simulink model "QPSK"  (R2020a)
settings: Solver=VariableStepAuto  StartTime=0.0  StopTime=200  RelTol=1e-3
libraries: simulink x7, dspsigops x2, commchan3 x1, dspstat3 x1, dspsrcs4 x1
settings Model: Creator=cxp10  LastModifiedBy=cxp10

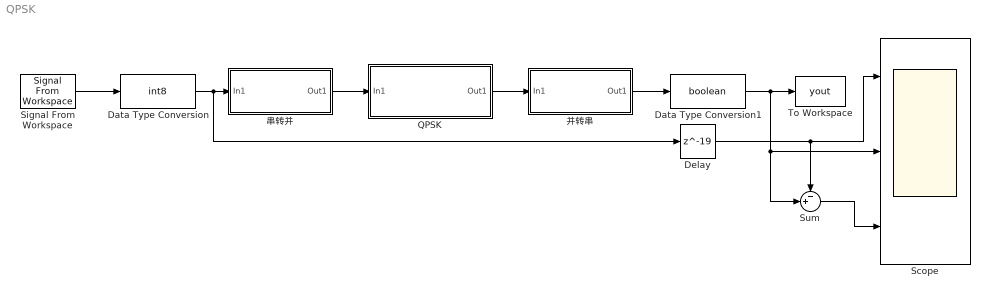
== system QPSK ==
  Data Type Conversion : DataTypeConversion  OutDataTypeStr=int8
  Data Type Conversion1 : DataTypeConversion  OutDataTypeStr=boolean
  Delay : Delay  DelayLength=19  InitialCondition=0  SampleTime=0.05
  QPSK : Subsystem
  Scope : Scope  NumInputPorts=3
  Signal From Workspace : dspsrcs4/Signal From Workspace  X=simin  Ts=0.05  nsamps=1  OutputAfterFinalValue=Setting to zero  ignoreOrWarnInputAndFrameLengths=off  OutputFrames=off
  Sum : Sum  Inputs=-+|
  To Workspace : ToWorkspace  VariableName=yout  SampleTime=-1
      settings: Save2DSignal=2-D array (concatenate along first dimension)
  串转并 : Subsystem
  并转串 : Subsystem
  wires:
  Data Type Conversion1/1 -> Sum/2, Scope/2, To Workspace/1
  Signal From Workspace/1 -> Data Type Conversion/1
  Sum/1 -> Scope/3
  并转串/1(Out1) -> Data Type Conversion1/1
  QPSK/1(Out1) -> 并转串/1(In1)
  串转并/1(Out1) -> QPSK/1(In1)
  Delay/1 -> Scope/1, Sum/1
  Data Type Conversion/1 -> 串转并/1(In1), Delay/1

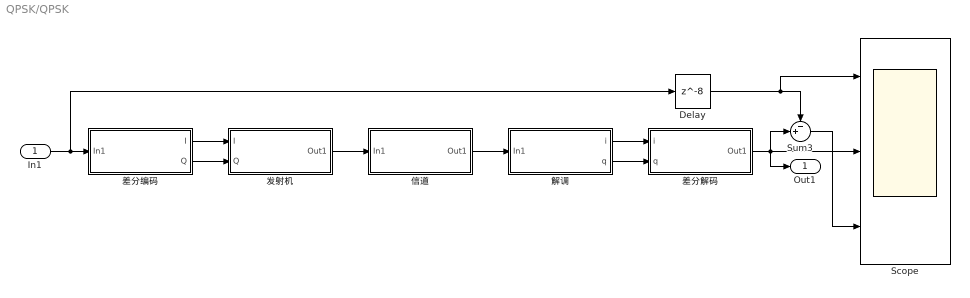
== system QPSK/QPSK ==
  In1 : Inport
  Delay : Delay  DelayLength=8  InitialCondition=0  SampleTime=0.1
  Scope : Scope  NumInputPorts=3
  Sum3 : Sum  Inputs=-+|
  信道 : Subsystem
  发射机 : Subsystem
  差分编码 : Subsystem
  差分解码 : Subsystem
  解调 : Subsystem
  Out1 : Outport
  wires:
  Delay/1 -> Sum3/1, Scope/1
  发射机/1(Out1) -> 信道/1(In1)
  解调/1(i) -> 差分解码/1(i)
  解调/2(q) -> 差分解码/2(q)
  信道/1(Out1) -> 解调/1(In1)
  Sum3/1 -> Scope/3
  差分编码/1(I) -> 发射机/1(I)
  差分编码/2(Q) -> 发射机/2(Q)
  In1/1 -> 差分编码/1(In1), Delay/1
  差分解码/1(Out1) -> Out1/1, Sum3/2, Scope/2

== system QPSK/串转并 ==
  In1 : Inport
  Delay : Delay  DelayLength=1  InitialCondition=0  SampleTime=0.05
  Delay1 : Delay  DelayLength=1  InitialCondition=0  SampleTime=0.1
  Gain : Gain  Gain=2
  Sum : Sum  Inputs=|++
  Out1 : Outport
  wires:
  Delay1/1 -> Out1/1
  Sum/1 -> Delay1/1
  In1/1 -> Sum/2, Delay/1
  Delay/1 -> Gain/1
  Gain/1 -> Sum/1

== system QPSK/并转串 ==
  In1 : Inport
  Counter Limited : simulink/Sources/Counter Limited  uplimit=1  tsamp=0.05
  Data Type Conversion : DataTypeConversion  OutDataTypeStr=fixdt(0,2,0)
  Extract Bits : simulink/Logic and Bit Operations/Extract Bits  bitsToExtract=Upper half  numBits=8  bitIdxRange=[0 7]  outScalingMode=Treat bit field as an integer
  Extract Bits1 : simulink/Logic and Bit Operations/Extract Bits  bitsToExtract=Lower half  numBits=8  bitIdxRange=[0 7]  outScalingMode=Treat bit field as an integer
  Switch : Switch  Criteria=u2 > Threshold
  Out1 : Outport
  wires:
  Extract Bits/1 -> Switch/3
  In1/1 -> Data Type Conversion/1
  Extract Bits1/1 -> Switch/1
  Data Type Conversion/1 -> Extract Bits1/1, Extract Bits/1
  Counter Limited/1 -> Switch/2
  Switch/1 -> Out1/1

== system QPSK/QPSK/信道 ==
  In1 : Inport
  AWGN Channel : commchan3/AWGN Channel  InputProcessing=Columns as channels (frame based)  seed=67  noiseMode="Signal to noise ratio  (SNR)"  EbNodB=10  EsNodB=10  SNRdB=5  bitsPerSym=1  Ps=0.0504  Tsym=1  variance=1
  Data Type Conversion : DataTypeConversion  OutDataTypeStr=double
  Data Type Conversion1 : DataTypeConversion
  Data Type Conversion2 : DataTypeConversion  OutDataTypeStr=fixdt(1,32,28)
  Mean : dspstat3/Mean  run=on  reset_popup=None  directionMode=Each column  dimension=1  roiEnable=off  roiType=Rectangles  roiPortion=Entire ROI  roiOutput=Individual statistics for each ROI  roiFlag=off  roundingMode=Floor  overflowMode=off  outputDataTypeStr=Inherit: Same as accumulator  outputMin=[]  outputMax=[]  outputLastDataTypeStr=Inherit: Same as accumulator
  Product : Product
  Scope1 : Scope
  Out1 : Outport
  wires:
  In1/1 -> Data Type Conversion/1
  AWGN Channel/1 -> Data Type Conversion2/1
  Data Type Conversion/1 -> Data Type Conversion1/1, AWGN Channel/1
  Product/1 -> Mean/1
  Data Type Conversion1/1 -> Product/2, Product/1
  Mean/1 -> Scope1/1
  Data Type Conversion2/1 -> Out1/1

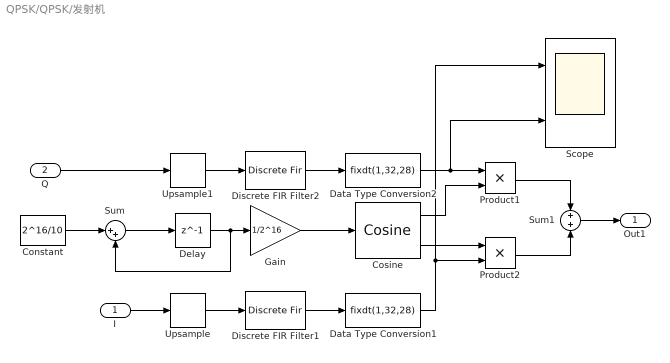
== system QPSK/QPSK/发射机 ==
  I : Inport
  Q : Inport  Port=2
  Constant : Constant  Value=2^16/10
  Cosine : simulink/Lookup Tables/Cosine  Formula=sin(2*pi*u) and cos(2*pi*u)  NumDataPoints=(2^16)+1  OutputWordLength=64  InternalRulePriority=Speed
      settings: SourceProductBaseCode=SL
  Data Type Conversion1 : DataTypeConversion  OutDataTypeStr=fixdt(1,32,28)
  Data Type Conversion2 : DataTypeConversion  OutDataTypeStr=fixdt(1,32,28)
  Delay : Delay  DelayLength=1  InitialCondition=0  SampleTime=0.01
  Discrete FIR Filter1 : DiscreteFir  Coefficients="[-0.0119566381847077\t-0.00554510890605436\t0.00241382573479933\t0.0111377436911783\t0.0196550101509641\t0.0268984171784200\t0.0318197882559029\t0.0335144832609033\t0.0313427539687735\t0.0250342434675171\t0.0147627477015526\t0.00118065713392810\t-0.0145939012931128\t-0.0310396234166703\t-0.0463415853998726\t-0.0585399944060724\t-0.0657057782491950\t-0.0661271775764019\t-0.0584895064408425\t-0.0420300071775653\t-0.0166513371647630\t0.0170194127981232\t0.0576344468660987\t0.103194189964349\t0.151177600592001\t0.198723997532092\t0.242851288478347\t0.280691625053822\t0.309723438717717\t0.327978774042235\t0.334206860938013\t0.327978774042235\t0.309723438717717\t0.280691625053822\t0.242851288478347\t0.198723997532092\t0.151177600592001\t0.103194189964349\t0.0576344468660987\t0.0170194127981232\t-0.0166513371647630\t-0.0420300071775653\t-0.0584895064408425\t-0.0661271775764019\t-0.0657057782491950\t-0.0585399944060724\t-0.0463415853998726\t-0.0310396234166703\t-0.0145939012931128\t0.00118065713392810\t0.0147627477015526\t0.0250342434675171\t0.0313427539687735\t0.0335144832609033\t0.0318197882559029\t0.0268984171784200\t0.0196550101509641\t0.0111377436911783\t0.00241382573479933\t-0.00554510890605436\t-0.0119566381847077]"
  Discrete FIR Filter2 : DiscreteFir  Coefficients="[-0.0119566381847077\t-0.00554510890605436\t0.00241382573479933\t0.0111377436911783\t0.0196550101509641\t0.0268984171784200\t0.0318197882559029\t0.0335144832609033\t0.0313427539687735\t0.0250342434675171\t0.0147627477015526\t0.00118065713392810\t-0.0145939012931128\t-0.0310396234166703\t-0.0463415853998726\t-0.0585399944060724\t-0.0657057782491950\t-0.0661271775764019\t-0.0584895064408425\t-0.0420300071775653\t-0.0166513371647630\t0.0170194127981232\t0.0576344468660987\t0.103194189964349\t0.151177600592001\t0.198723997532092\t0.242851288478347\t0.280691625053822\t0.309723438717717\t0.327978774042235\t0.334206860938013\t0.327978774042235\t0.309723438717717\t0.280691625053822\t0.242851288478347\t0.198723997532092\t0.151177600592001\t0.103194189964349\t0.0576344468660987\t0.0170194127981232\t-0.0166513371647630\t-0.0420300071775653\t-0.0584895064408425\t-0.0661271775764019\t-0.0657057782491950\t-0.0585399944060724\t-0.0463415853998726\t-0.0310396234166703\t-0.0145939012931128\t0.00118065713392810\t0.0147627477015526\t0.0250342434675171\t0.0313427539687735\t0.0335144832609033\t0.0318197882559029\t0.0268984171784200\t0.0196550101509641\t0.0111377436911783\t0.00241382573479933\t-0.00554510890605436\t-0.0119566381847077]"
  Gain : Gain  Gain=1/2^16
  Product1 : Product  OutDataTypeStr=fixdt(1,32,28)
  Product2 : Product  OutDataTypeStr=fixdt(1,32,28)
  Scope : Scope  NumInputPorts=2
  Sum : Sum  Inputs=|++  OutMin=[0]  OutMax=[2^16-1]  OutDataTypeStr=fixdt(0,32,16)
  Sum1 : Sum  Inputs=+|+
  Upsample : dspsigops/Upsample  N=10  phase=0  RateOptions=Allow multirate processing  ic=0  mode=Unused parameter value
  Upsample1 : dspsigops/Upsample  N=10  phase=0  RateOptions=Allow multirate processing  ic=0  mode=Unused parameter value
  Out1 : Outport
  wires:
  Constant/1 -> Sum/1
  Upsample1/1 -> Discrete FIR Filter2/1
  Product1/1 -> Sum1/1
  Cosine/2 -> Product2/1
  Product2/1 -> Sum1/2
  Sum/1 -> Delay/1
  Cosine/1 -> Product1/2
  Q/1 -> Upsample1/1
  Sum1/1 -> Out1/1
  Discrete FIR Filter2/1 -> Data Type Conversion2/1
  Discrete FIR Filter1/1 -> Data Type Conversion1/1
  Upsample/1 -> Discrete FIR Filter1/1
  I/1 -> Upsample/1
  Gain/1 -> Cosine/1
  Data Type Conversion1/1 -> Scope/1, Product2/2
  Data Type Conversion2/1 -> Scope/2, Product1/1
  Delay/1 -> Gain/1, Sum/2

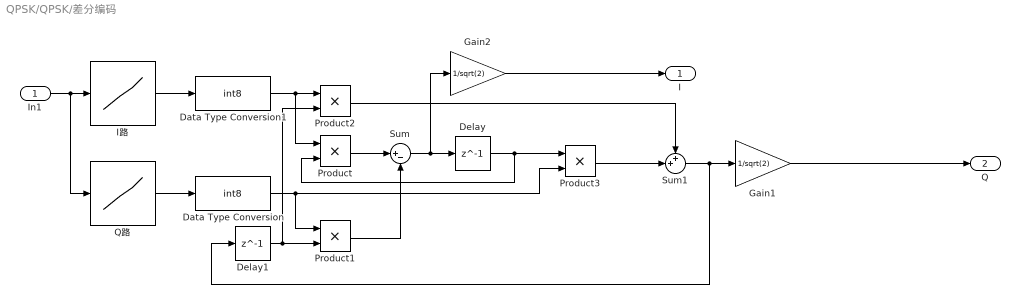
== system QPSK/QPSK/差分编码 ==
  In1 : Inport
  Data Type Conversion : DataTypeConversion  OutDataTypeStr=int8
  Data Type Conversion1 : DataTypeConversion  OutDataTypeStr=int8
  Delay : Delay  DelayLength=1  InitialCondition=1  SampleTime=0.1
  Delay1 : Delay  DelayLength=1  InitialCondition=1  SampleTime=0.1
  Gain1 : Gain  Gain=1/sqrt(2)  OutDataTypeStr=fixdt(1,32,28)
  Gain2 : Gain  Gain=1/sqrt(2)  OutDataTypeStr=fixdt(1,32,28)
  I路 : Lookup_n-D  NumberOfTableDimensions=1  BreakpointsForDimension1=[0:3]  BreakpointsForDimension2=[0:3]  Table=[1 0 0 -1]  ExtrapMethod=Clip  InternalRulePriority=Speed  RndMeth=Simplest  InputSameDT=on
  Product{,1..3} (4 alike) : Product  OutDataTypeStr=int8
  Q路 : Lookup_n-D  NumberOfTableDimensions=1  BreakpointsForDimension1=[0:3]  BreakpointsForDimension2=[0:3]  Table=[0 1 -1 0]  ExtrapMethod=Clip  InternalRulePriority=Speed  RndMeth=Simplest  InputSameDT=on
  Sum : Sum  Inputs=|+-
  Sum1 : Sum  Inputs=++|
  I : Outport
  Q : Outport  Port=2
  wires:
  Product1/1 -> Sum/2
  Gain2/1 -> I/1
  Gain1/1 -> Q/1
  Product/1 -> Sum/1
  In1/1 -> I路/1, Q路/1
  Product2/1 -> Sum1/1
  Product3/1 -> Sum1/2
  Q路/1 -> Data Type Conversion/1
  I路/1 -> Data Type Conversion1/1
  Data Type Conversion1/1 -> Product2/1, Product/1
  Data Type Conversion/1 -> Product3/2, Product1/1
  Delay/1 -> Product3/1, Product/2
  Sum/1 -> Gain2/1, Delay/1
  Delay1/1 -> Product1/2, Product2/2
  Sum1/1 -> Gain1/1, Delay1/1

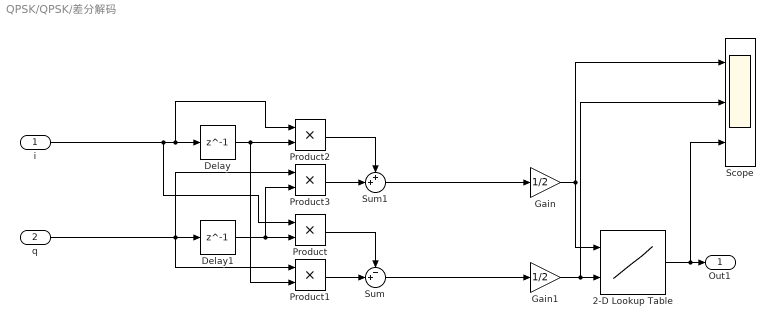
== system QPSK/QPSK/差分解码 ==
  i : Inport
  q : Inport  Port=2
  2-D Lookup Table : Lookup_n-D  BreakpointsForDimension1=[-1 0 1]  BreakpointsForDimension2=[-1 0 1]  Table=[0 3 0; 2 0 1; 0 0 0]  ExtrapMethod=Clip  InternalRulePriority=Speed  RndMeth=Simplest  InputSameDT=on
  Delay : Delay  DelayLength=1  InitialCondition=0  SampleTime=0.1
  Delay1 : Delay  DelayLength=1  InitialCondition=0  SampleTime=0.1
  Gain : Gain  Gain=1/2  OutDataTypeStr=fixdt(1,32,28)
  Gain1 : Gain  Gain=1/2  OutDataTypeStr=fixdt(1,32,28)
  Product{,1..3} (4 alike) : Product  OutDataTypeStr=fixdt(1,32,28)
  Scope : Scope  NumInputPorts=3
  Sum : Sum  Inputs=-+|  OutDataTypeStr=fixdt(1,32,28)
  Sum1 : Sum  Inputs=++|  OutDataTypeStr=fixdt(1,32,28)
  Out1 : Outport
  wires:
  Gain/1 -> Scope/1, 2-D Lookup Table/1
  Product1/1 -> Sum/2
  Product/1 -> Sum/1
  Product2/1 -> Sum1/1
  Product3/1 -> Sum1/2
  Gain1/1 -> Scope/2, 2-D Lookup Table/2
  2-D Lookup Table/1 -> Scope/3, Out1/1
  q/1 -> Delay1/1, Product1/1, Product3/1
  i/1 -> Product2/1, Delay/1, Product/1
  Delay/1 -> Product2/2, Product1/2
  Delay1/1 -> Product/2, Product3/2
  Sum1/1 -> Gain/1
  Sum/1 -> Gain1/1

== system QPSK/QPSK/解调 ==
  In1 : Inport
  Delay2 : Delay  DelayLength=1  InitialCondition=0  SampleTime=0.01
  Gain1 : Gain  Gain=5/sqrt(2)  OutDataTypeStr=fixdt(1,32,28)
  Scope : Scope  NumInputPorts=3
  位同步 : Subsystem
  载波同步 : Subsystem
  i : Outport
  q : Outport  Port=2
  wires:
  位同步/2(Q) -> q/1
  载波同步/2(q) -> 位同步/2(q), Scope/3
  载波同步/1(i) -> 位同步/1(i), Scope/2
  Delay2/1 -> Gain1/1
  In1/1 -> Delay2/1
  位同步/1(I) -> i/1
  Gain1/1 -> Scope/1, 载波同步/1(In1)

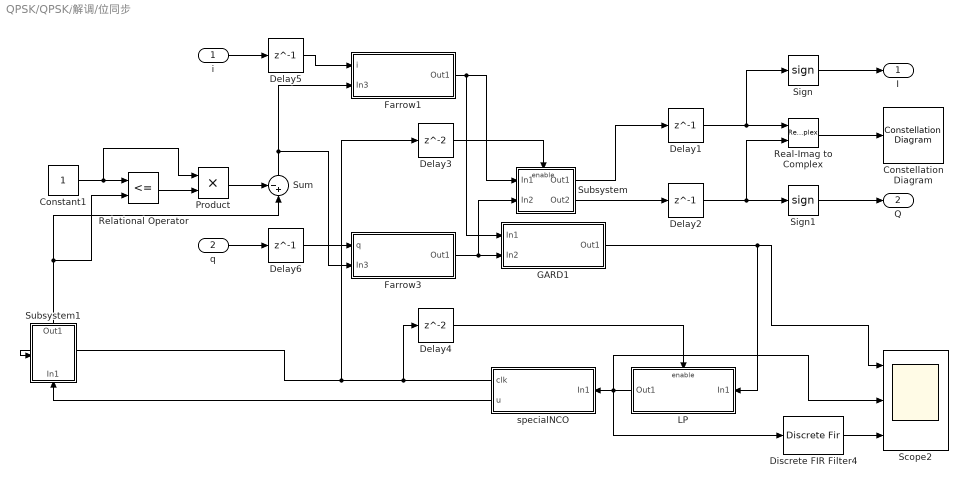
== system QPSK/QPSK/解调/位同步 ==
  i : Inport
  q : Inport  Port=2
  Constant1 : Constant  OutDataTypeStr=fixdt(1,32,28)  SampleTime=0.01
  Constellation Diagram : ConstellationDiagram
  Delay1 : Delay  DelayLength=1  InitialCondition=0  SampleTime=0.1
  Delay2 : Delay  DelayLength=1  InitialCondition=0  SampleTime=0.1
  Delay3 : Delay  InitialCondition=0
  Delay4 : Delay  InitialCondition=0
  Delay5 : Delay  DelayLength=1  InitialCondition=0  SampleTime=0.01
  Delay6 : Delay  DelayLength=1  InitialCondition=0  SampleTime=0.01
  Discrete FIR Filter4 : DiscreteFir  Coefficients="[5.38827670327720e-05\t8.37859864059126e-06\t9.02577071280919e-06\t9.70599515144445e-06\t1.04165818557214e-05\t1.11621497031896e-05\t1.19399905979190e-05\t1.27547662205456e-05\t1.36038280216497e-05\t1.44919424768979e-05\t1.54165002359471e-05\t1.63821647738810e-05\t1.73863448370645e-05\t1.84338552877666e-05\t1.95220392829791e-05\t2.06555805408248e-05\t2.18322698177188e-05\t2.30558422383026e-05\t2.43269378472256e-05\t2.56438783973424e-05\t2.70139194785259e-05\t2.84325674352020e-05\t2.99013001451981e-05\t3.14273576150905e-05\t3.30048430841328e-05\t3.46380754777013e-05\t3.63271213027826e-05\t3.80773652938778e-05\t3.98849018394236e-05\t4.17539156292012e-05\t4.36830329961517e-05\t4.56781471467015e-05\t4.77366900846824e-05\t4.98628301063512e-05\t5.20540085491405e-05\t5.43152490247501e-05\t5.66456038712473e-05\t5.90491252349792e-05\t6.15249958158559e-05\t6.40756749798356e-05\t6.67003989259873e-05\t6.94040934711277e-05\t7.21842036194296e-05\t7.50467729337769e-05\t7.79894707634970e-05\t8.10163281991232e-05\t8.41252815914495e-05\t8.73216363738031e-05\t9.06029889739106e-05\t9.39743974468708e-05\t9.74342060955591e-05\t0.000100987692375075\t0.000104632192107747\t0.000108372281681474\t0.000112206342467372\t0.000116139266468525\t0.000120169404871481\t0.000124301052804280\t0.000128532823220613\t0.000132869575729040\t0.000137309181029465\t0.000141856789010187\t0.000146509847117926\t0.000151273286674838\t0.000156145642667454\t0.000161132018009352\t0.000166230083764592\t0.000171444733398769\t0.000176773605960749\t0.000182221612661642\t0.000187786593150612\t0.000193473629150883\t0.000199280488718983\t0.000205211685132340\t0.000211265398500019\t0.000217446507607164\t0.000223752761217449\t0.000230188784560116\t0.000236752520818625\t0.000243448735435774\t0.000250274983037235\t0.000257236019535067\t0.000264330100506618\t0.000271561990243754\t0.000278929355274878\t0.000286436890265331\t0.000294082033792734\t0.000301869596439394\t0.000309797345205324\t0.000317870189475281\t0.000326085384863677\t0.000334447075689439\t0.000342952903655544\t0.000351607352631286\t0.000360407616665803\t0.000369358318123430\t0.000378456801352178\t0.000387707364382725\t0.000397108082112494\t0.000406662934343845\t0.000416369204580440\t0.000426230755104286\t0.000436245388557304\t0.000446417742153065\t0.000456744884181980\t0.000467231199909950\t0.000477873972464166\t0.000488677251350832\t0.000499637440376430\t0.000510758673367827\t0.000522038396887917\t0.000533480280401991\t0.000545080769398471\t0.000556844103994101\t0.000568766185736806\t0.000580850432672023\t0.000593095234683480\t0.000605503378253917\t0.000618072781238363\t0.000630806222575761\t0.000643700780350444\t0.000656760471832712\t0.000669982400586430\t0.000683370025829815\t0.000696918573098365\t0.000710630926905871\t0.000724503829445785\t0.000738540917568113\t0.000752737001090627\t0.000767094386499337\t0.000781610766006477\t0.000796290631539730\t0.000811128092858480\t0.000826127681412666\t0.000841289250929616\t0.000856610300748781\t0.000872091884416860\t0.000887732449192652\t0.000903528018728126\t0.000919479373359454\t0.000935581446470775\t0.000951837298855666\t0.000968244039667702\t0.000984807285270455\t0.00100152517468790\t0.00101840099564402\t0.00103542695598586\t0.00105259888833481\t0.00106990529758374\t0.00108734964897944\t0.00110494267566542\t0.00112270934980982\t0.00114063129213466\t0.00115859990752069\t0.00117680222888921\t0.00119509959387189\t0.00121353986073303\t0.00123211546656185\t0.00125082134371779\t0.00126965953442028\t0.00128862434940582\t0.00130771774074139\t0.00132693385136779\t0.00134627449466985\t0.00136573389331197\t0.00138531384301694\t0.00140500830367386\t0.00142481894640172\t0.00144473975340373\t0.00146477179813887\t0.00148491072277744\t0.00150515201712332\t0.00152550251281669\t0.00154594432004887\t0.00156648817916740\t0.00158713046774516\t0.00160785883937208\t0.00162867840978680\t0.00164958598216596\t0.00167058052426799\t0.00169165284490608\t0.00171280423850651\t0.00173403000161468\t0.00175533174791612\t0.00177670178930184\t0.00179813963787842\t0.00181963802898036\t0.00184119812822650\t0.00186281437153346\t0.00188448678592134\t0.00190620967124911\t0.00192798028738096\t0.00194979411140008\t0.00197164956662192\t0.00199354018589733\t0.00201546789161710\t0.00203742463061031\t0.00205941027148300\t0.00208141816454080\t0.00210344802294037\t0.00212549178019049\t0.00214754993849286\t0.00216961587770786\t0.00219168966688694\t0.00221376332118668\t0.00223583683848542\t0.00225790312180091\t0.00227996159306796\t0.00230200480313444\t0.00232403181786743\t0.00234603631036743\t0.00236801777706385\t0.00238996920742478\t0.00241189033720393\t0.00243377280023632\t0.00245561659728671\t0.00247741441458659\t0.00249916562476833\t0.00252086247707472\t0.00254250471250362\t0.00256408444650458\t0.00258560151102332\t0.00260704842123784\t0.00262842494172428\t0.00264972299974808\t0.00267094199109233\t0.00269207461389840\t0.00271312023792777\t0.00273407126085464\t0.00275492724121749\t0.00277568079319803\t0.00279633128757952\t0.00281687073335238\t0.00283729896652871\t0.00285760864563827\t0.00287779930865078\t0.00289786332489527\t0.00291780003374124\t0.00293760134158108\t0.00295726700042838\t0.00297678944775037\t0.00299616850302645\t0.00301539634921388\t0.00303447287903666\t0.00305339092046008\t0.00307215012960474\t0.00309074294525690\t0.00310916914923290\t0.00312742099521662\t0.00314549848505173\t0.00316339462896414\t0.00318110881202524\t0.00319863347580294\t0.00321596813726239\t0.00323310586877002\t0.00325004654568439\t0.00326678292509291\t0.00328331562337832\t0.00329963761639421\t0.00331574889348412\t0.00333164194876551\t0.00334731729334170\t0.00336276794775731\t0.00337799391711069\t0.00339298833367161\t0.00340775154497468\t0.00342227577383967\t0.00343656199966569\t0.00345060427242355\t0.00346440245671541\t0.00347795086958273\t0.00349124911036735\t0.00350429126057300\t0.00351707814873492\t0.00352960351071997\t0.00354186762564742\t0.00355386316841616\t0.00356559141606362\t0.00357704675895919\t0.00358823039438686\t0.00359913555335254\t0.00360976414503881\t0.00362011126863201\t0.00363017742507951\t0.00363995506211021\t0.00364944695575173\t0.00365864686422917\t0.00366755392779621\t0.00367616707788512\t0.00368448516912521\t0.00369250555052204\t0.00370022882430508\t0.00370764908188711\t0.00371476694754616\t0.00372157637874722\t0.00372808046376311\t0.00373427584403981\t0.00374016638993305\t0.00374574619888750\t0.00375101445240137\t0.00375596347238067\t0.00376059842158154\t0.00376492136939815\t0.00376893584053243\t0.00377262402091522\t0.00377598540971720\t0.00377905127976721\t0.00378177794701704\t0.00378419317618726\t0.00378628656092737\t0.00378805733185340\t0.00378950843311406\t0.00379063573696286\t0.00379144285830933\t0.00379192563658652\t0.00379208785170762\t0.00379192563658652\t0.00379144285830933\t0.00379063573696286\t0.00378950843311406\t0.00378805733185340\t0.00378628656092737\t0.00378419317618726\t0.00378177794701704\t0.00377905127976721\t0.00377598540971720\t0.00377262402091522\t0.00376893584053243\t0.00376492136939815\t0.00376059842158154\t0.00375596347238067\t0.00375101445240137\t0.00374574619888750\t0.00374016638993305\t0.00373427584403981\t0.00372808046376311\t0.00372157637874722\t0.00371476694754616\t0.00370764908188711\t0.00370022882430508\t0.00369250555052204\t0.00368448516912521\t0.00367616707788512\t0.00366755392779621\t0.00365864686422917\t0.00364944695575173\t0.00363995506211021\t0.00363017742507951\t0.00362011126863201\t0.00360976414503881\t0.00359913555335254\t0.00358823039438686\t0.00357704675895919\t0.00356559141606362\t0.00355386316841616\t0.00354186762564742\t0.00352960351071997\t0.00351707814873492\t0.00350429126057300\t0.00349124911036735\t0.00347795086958273\t0.00346440245671541\t0.00345060427242355\t0.00343656199966569\t0.00342227577383967\t0.00340775154497468\t0.00339298833367161\t0.00337799391711069\t0.00336276794775731\t0.00334731729334170\t0.00333164194876551\t0.00331574889348412\t0.00329963761639421\t0.00328331562337832\t0.00326678292509291\t0.00325004654568439\t0.00323310586877002\t0.00321596813726239\t0.00319863347580294\t0.00318110881202524\t0.00316339462896414\t0.00314549848505173\t0.00312742099521662\t0.00310916914923290\t0.00309074294525690\t0.00307215012960474\t0.00305339092046008\t0.00303447287903666\t0.00301539634921388\t0.00299616850302645\t0.00297678944775037\t0.00295726700042838\t0.00293760134158108\t0.00291780003374124\t0.00289786332489527\t0.00287779930865078\t0.00285760864563827\t0.00283729896652871\t0.00281687073335238\t0.00279633128757952\t0.00277568079319803\t0.00275492724121749\t0.00273407126085464\t0.00271312023792777\t0.00269207461389840\t0.00267094199109233\t0.00264972299974808\t0.00262842494172428\t0.00260704842123784\t0.00258560151102332\t0.00256408444650458\t0.00254250471250362\t0.00252086247707472\t0.00249916562476833\t0.00247741441458659\t0.00245561659728671\t0.00243377280023632\t0.00241189033720393\t0.00238996920742478\t0.00236801777706385\t0.00234603631036743\t0.00232403181786743\t0.00230200480313444\t0.00227996159306796\t0.00225790312180091\t0.00223583683848542\t0.00221376332118668\t0.00219168966688694\t0.00216961587770786\t0.00214754993849286\t0.00212549178019049\t0.00210344802294037\t0.00208141816454080\t0.00205941027148300\t0.00203742463061031\t0.00201546789161710\t0.00199354018589733\t0.00197164956662192\t0.00194979411140008\t0.00192798028738096\t0.00190620967124911\t0.00188448678592134\t0.00186281437153346\t0.00184119812822650\t0.00181963802898036\t0.00179813963787842\t0.00177670178930184\t0.00175533174791612\t0.00173403000161468\t0.00171280423850651\t0.00169165284490608\t0.00167058052426799\t0.00164958598216596\t0.00162867840978680\t0.00160785883937208\t0.00158713046774516\t0.00156648817916740\t0.00154594432004887\t0.00152550251281669\t0.00150515201712332\t0.00148491072277744\t0.00146477179813887\t0.00144473975340373\t0.00142481894640172\t0.00140500830367386\t0.00138531384301694\t0.00136573389331197\t0.00134627449466985\t0.00132693385136779\t0.00130771774074139\t0.00128862434940582\t0.00126965953442028\t0.00125082134371779\t0.00123211546656185\t0.00121353986073303\t0.00119509959387189\t0.00117680222888921\t0.00115859990752069\t0.00114063129213466\t0.00112270934980982\t0.00110494267566542\t0.00108734964897944\t0.00106990529758374\t0.00105259888833481\t0.00103542695598586\t0.00101840099564402\t0.00100152517468790\t0.000984807285270455\t0.000968244039667702\t0.000951837298855666\t0.000935581446470775\t0.000919479373359454\t0.000903528018728126\t0.000887732449192652\t0.000872091884416860\t0.000856610300748781\t0.000841289250929616\t0.000826127681412666\t0.000811128092858480\t0.000796290631539730\t0.000781610766006477\t0.000767094386499337\t0.000752737001090627\t0.000738540917568113\t0.000724503829445785\t0.000710630926905871\t0.000696918573098365\t0.000683370025829815\t0.000669982400586430\t0.000656760471832712\t0.000643700780350444\t0.000630806222575761\t0.000618072781238363\t0.000605503378253917\t0.000593095234683480\t0.000580850432672023\t0.000568766185736806\t0.000556844103994101\t0.000545080769398471\t0.000533480280401991\t0.000522038396887917\t0.000510758673367827\t0.000499637440376430\t0.000488677251350832\t0.000477873972464166\t0.000467231199909950\t0.000456744884181980\t0.000446417742153065\t0.000436245388557304\t0.000426230755104286\t0.000416369204580440\t0.000406662934343845\t0.000397108082112494\t0.000387707364382725\t0.000378456801352178\t0.000369358318123430\t0.000360407616665803\t0.000351607352631286\t0.000342952903655544\t0.000334447075689439\t0.000326085384863677\t0.000317870189475281\t0.000309797345205324\t0.000301869596439394\t0.000294082033792734\t0.000286436890265331\t0.000278929355274878\t0.000271561990243754\t0.000264330100506618\t0.000257236019535067\t0.000250274983037235\t0.000243448735435774\t0.000236752520818625\t0.000230188784560116\t0.000223752761217449\t0.000217446507607164\t0.000211265398500019\t0.000205211685132340\t0.000199280488718983\t0.000193473629150883\t0.000187786593150612\t0.000182221612661642\t0.000176773605960749\t0.000171444733398769\t0.000166230083764592\t0.000161132018009352\t0.000156145642667454\t0.000151273286674838\t0.000146509847117926\t0.000141856789010187\t0.000137309181029465\t0.000132869575729040\t0.000128532823220613\t0.000124301052804280\t0.000120169404871481\t0.000116139266468525\t0.000112206342467372\t0.000108372281681474\t0.000104632192107747\t0.000100987692375075\t9.74342060955591e-05\t9.39743974468708e-05\t9.06029889739106e-05\t8.73216363738031e-05\t8.41252815914495e-05\t8.10163281991232e-05\t7.79894707634970e-05\t7.50467729337769e-05\t7.21842036194296e-05\t6.94040934711277e-05\t6.67003989259873e-05\t6.40756749798356e-05\t6.15249958158559e-05\t5.90491252349792e-05\t5.66456038712473e-05\t5.43152490247501e-05\t5.20540085491405e-05\t4.98628301063512e-05\t4.77366900846824e-05\t4.56781471467015e-05\t4.36830329961517e-05\t4.17539156292012e-05\t3.98849018394236e-05\t3.80773652938778e-05\t3.63271213027826e-05\t3.46380754777013e-05\t3.30048430841328e-05\t3.14273576150905e-05\t2.99013001451981e-05\t2.84325674352020e-05\t2.70139194785259e-05\t2.56438783973424e-05\t2.43269378472256e-05\t2.30558422383026e-05\t2.18322698177188e-05\t2.06555805408248e-05\t1.95220392829791e-05\t1.84338552877666e-05\t1.73863448370645e-05\t1.63821647738810e-05\t1.54165002359471e-05\t1.44919424768979e-05\t1.36038280216497e-05\t1.27547662205456e-05\t1.19399905979190e-05\t1.11621497031896e-05\t1.04165818557214e-05\t9.70599515144445e-06\t9.02577071280919e-06\t8.37859864059126e-06\t5.38827670327720e-05]"
  Farrow1 : Subsystem
  Farrow3 : Subsystem
  GARD1 : Subsystem
  LP : Subsystem
  Product : Product
  Real-Imag to Complex : RealImagToComplex
  Relational Operator : RelationalOperator  Operator=<=  OutDataTypeStr=boolean  RndMeth=Simplest
  Scope2 : Scope  NumInputPorts=3
  Sign : Signum
  Sign1 : Signum
  Subsystem : Subsystem
  Subsystem1 : Subsystem
  Sum : Sum  Inputs=-+|  OutDataTypeStr=fixdt(1,32,28)
  specialNCO : Subsystem
  I : Outport
  Q : Outport  Port=2
  wires:
  Real-Imag to Complex/1 -> Constellation Diagram/1
  Sign/1 -> I/1
  Sign1/1 -> Q/1
  Discrete FIR Filter4/1 -> Scope2/3
  Product/1 -> Sum/1
  Relational Operator/1 -> Product/2
  Farrow1/1(Out1) -> GARD1/1(In1), Subsystem/1(In1)
  Delay6/1 -> Farrow3/1(q)
  Delay5/1 -> Farrow1/1(i)
  specialNCO/1(clk) -> Delay3/1, Subsystem1/Enable, Delay4/1
  q/1 -> Delay6/1
  i/1 -> Delay5/1
  Subsystem/1(Out1) -> Delay1/1
  Sum/1 -> Farrow1/2(In3), Farrow3/2(In3)
  Delay4/1 -> LP/Enable
  Subsystem1/1(Out1) -> Sum/2, Relational Operator/2
  Delay3/1 -> Subsystem/Enable
  LP/1(Out1) -> Scope2/2, Discrete FIR Filter4/1, specialNCO/1(In1)
  specialNCO/2(u) -> Subsystem1/1(In1)
  Subsystem/2(Out2) -> Delay2/1
  Delay1/1 -> Sign/1, Real-Imag to Complex/1
  Delay2/1 -> Sign1/1, Real-Imag to Complex/2
  Constant1/1 -> Relational Operator/1, Product/1
  GARD1/1(Out1) -> Scope2/1, LP/1(In1)
  Farrow3/1(Out1) -> GARD1/2(In2), Subsystem/2(In2)

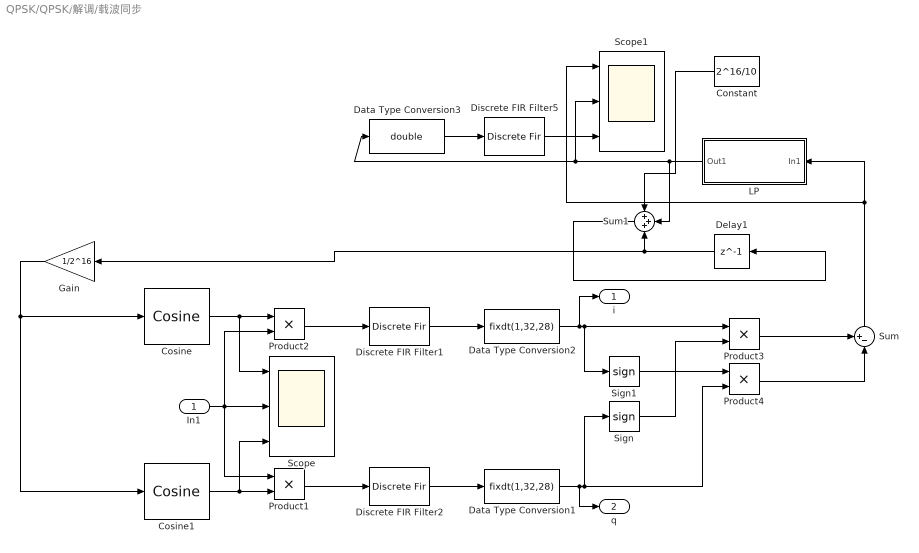
== system QPSK/QPSK/解调/载波同步 ==
  In1 : Inport
  Constant : Constant  Value=2^16/10
  Cosine : simulink/Lookup Tables/Cosine  Formula=cos(2*pi*u)  NumDataPoints=(2^16)+1  OutputWordLength=64  InternalRulePriority=Speed
      settings: SourceProductBaseCode=SL
  Cosine1 : simulink/Lookup Tables/Cosine  Formula=sin(2*pi*u)  NumDataPoints=(2^16)+1  OutputWordLength=64  InternalRulePriority=Speed
      settings: SourceProductBaseCode=SL
  Data Type Conversion1 : DataTypeConversion  OutDataTypeStr=fixdt(1,32,28)
  Data Type Conversion2 : DataTypeConversion  OutDataTypeStr=fixdt(1,32,28)
  Data Type Conversion3 : DataTypeConversion  OutDataTypeStr=double
  Delay1 : Delay  DelayLength=1  InitialCondition=0  SampleTime=0.01
  Discrete FIR Filter1 : DiscreteFir  Coefficients="[-0.0119566381847077\t-0.00554510890605436\t0.00241382573479933\t0.0111377436911783\t0.0196550101509641\t0.0268984171784200\t0.0318197882559029\t0.0335144832609033\t0.0313427539687735\t0.0250342434675171\t0.0147627477015526\t0.00118065713392810\t-0.0145939012931128\t-0.0310396234166703\t-0.0463415853998726\t-0.0585399944060724\t-0.0657057782491950\t-0.0661271775764019\t-0.0584895064408425\t-0.0420300071775653\t-0.0166513371647630\t0.0170194127981232\t0.0576344468660987\t0.103194189964349\t0.151177600592001\t0.198723997532092\t0.242851288478347\t0.280691625053822\t0.309723438717717\t0.327978774042235\t0.334206860938013\t0.327978774042235\t0.309723438717717\t0.280691625053822\t0.242851288478347\t0.198723997532092\t0.151177600592001\t0.103194189964349\t0.0576344468660987\t0.0170194127981232\t-0.0166513371647630\t-0.0420300071775653\t-0.0584895064408425\t-0.0661271775764019\t-0.0657057782491950\t-0.0585399944060724\t-0.0463415853998726\t-0.0310396234166703\t-0.0145939012931128\t0.00118065713392810\t0.0147627477015526\t0.0250342434675171\t0.0313427539687735\t0.0335144832609033\t0.0318197882559029\t0.0268984171784200\t0.0196550101509641\t0.0111377436911783\t0.00241382573479933\t-0.00554510890605436\t-0.0119566381847077]"
  Discrete FIR Filter2 : DiscreteFir  Coefficients="[-0.0119566381847077\t-0.00554510890605436\t0.00241382573479933\t0.0111377436911783\t0.0196550101509641\t0.0268984171784200\t0.0318197882559029\t0.0335144832609033\t0.0313427539687735\t0.0250342434675171\t0.0147627477015526\t0.00118065713392810\t-0.0145939012931128\t-0.0310396234166703\t-0.0463415853998726\t-0.0585399944060724\t-0.0657057782491950\t-0.0661271775764019\t-0.0584895064408425\t-0.0420300071775653\t-0.0166513371647630\t0.0170194127981232\t0.0576344468660987\t0.103194189964349\t0.151177600592001\t0.198723997532092\t0.242851288478347\t0.280691625053822\t0.309723438717717\t0.327978774042235\t0.334206860938013\t0.327978774042235\t0.309723438717717\t0.280691625053822\t0.242851288478347\t0.198723997532092\t0.151177600592001\t0.103194189964349\t0.0576344468660987\t0.0170194127981232\t-0.0166513371647630\t-0.0420300071775653\t-0.0584895064408425\t-0.0661271775764019\t-0.0657057782491950\t-0.0585399944060724\t-0.0463415853998726\t-0.0310396234166703\t-0.0145939012931128\t0.00118065713392810\t0.0147627477015526\t0.0250342434675171\t0.0313427539687735\t0.0335144832609033\t0.0318197882559029\t0.0268984171784200\t0.0196550101509641\t0.0111377436911783\t0.00241382573479933\t-0.00554510890605436\t-0.0119566381847077]"
  Discrete FIR Filter5 : DiscreteFir  Coefficients="[-0.0119566381847077\t-0.00554510890605436\t0.00241382573479933\t0.0111377436911783\t0.0196550101509641\t0.0268984171784200\t0.0318197882559029\t0.0335144832609033\t0.0313427539687735\t0.0250342434675171\t0.0147627477015526\t0.00118065713392810\t-0.0145939012931128\t-0.0310396234166703\t-0.0463415853998726\t-0.0585399944060724\t-0.0657057782491950\t-0.0661271775764019\t-0.0584895064408425\t-0.0420300071775653\t-0.0166513371647630\t0.0170194127981232\t0.0576344468660987\t0.103194189964349\t0.151177600592001\t0.198723997532092\t0.242851288478347\t0.280691625053822\t0.309723438717717\t0.327978774042235\t0.334206860938013\t0.327978774042235\t0.309723438717717\t0.280691625053822\t0.242851288478347\t0.198723997532092\t0.151177600592001\t0.103194189964349\t0.0576344468660987\t0.0170194127981232\t-0.0166513371647630\t-0.0420300071775653\t-0.0584895064408425\t-0.0661271775764019\t-0.0657057782491950\t-0.0585399944060724\t-0.0463415853998726\t-0.0310396234166703\t-0.0145939012931128\t0.00118065713392810\t0.0147627477015526\t0.0250342434675171\t0.0313427539687735\t0.0335144832609033\t0.0318197882559029\t0.0268984171784200\t0.0196550101509641\t0.0111377436911783\t0.00241382573479933\t-0.00554510890605436\t-0.0119566381847077]"
  Gain : Gain  Gain=1/2^16
  LP : Subsystem
  Product{1..4} (4 alike) : Product  OutDataTypeStr=fixdt(1,32,28)
  Scope : Scope  NumInputPorts=3
  Scope1 : Scope  NumInputPorts=3
  Sign : Signum
  Sign1 : Signum
  Sum : Sum  Inputs=+-|
  Sum1 : Sum  Inputs=+++  OutMin=[0]  OutMax=[2^16-1]  OutDataTypeStr=fixdt(1,32,15)
  i : Outport
  q : Outport  Port=2
  wires:
  Sum1/1 -> Delay1/1
  Discrete FIR Filter5/1 -> Scope1/3
  Product3/1 -> Sum/1
  Product4/1 -> Sum/2
  Discrete FIR Filter1/1 -> Data Type Conversion2/1
  Constant/1 -> Sum1/1
  Product2/1 -> Discrete FIR Filter1/1
  Discrete FIR Filter2/1 -> Data Type Conversion1/1
  Product1/1 -> Discrete FIR Filter2/1
  Data Type Conversion3/1 -> Discrete FIR Filter5/1
  Sign1/1 -> Product4/1
  Sign/1 -> Product3/2
  Sum/1 -> LP/1(In1), Scope1/1
  Gain/1 -> Cosine/1, Cosine1/1
  Data Type Conversion1/1 -> Sign/1, Product4/2, q/1
  In1/1 -> Scope/2, Product1/1, Product2/2
  Cosine1/1 -> Product1/2, Scope/3
  Delay1/1 -> Sum1/3, Gain/1
  Cosine/1 -> Product2/1, Scope/1
  LP/1(Out1) -> Sum1/2, Scope1/2, Data Type Conversion3/1
  Data Type Conversion2/1 -> Product3/1, Sign1/1, i/1

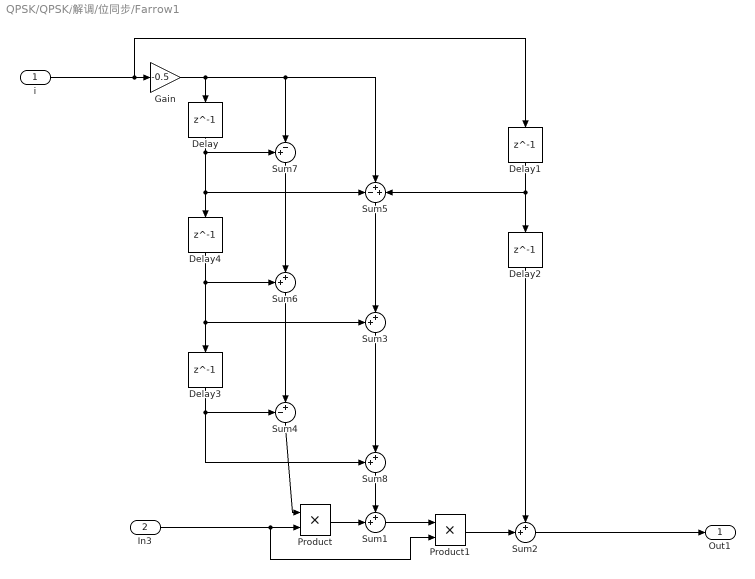
== system QPSK/QPSK/解调/位同步/Farrow1 ==
  i : Inport
  In3 : Inport  Port=2
  Delay{,1..4} (5 alike) : Delay  DelayLength=1  InitialCondition=0
  Gain : Gain  Gain=-0.5  OutDataTypeStr=fixdt(1,32,28)
  Product : Product  OutDataTypeStr=fixdt(1,32,28)
  Product1 : Product  OutDataTypeStr=fixdt(1,32,28)
  Sum{1,3,6,8} (4 alike) : Sum  Inputs=++|
  Sum2 : Sum  Inputs=++|  OutDataTypeStr=fixdt(1,32,28)
  Sum4 : Sum  Inputs=-+|
  Sum5 : Sum  Inputs=-++
  Sum7 : Sum  Inputs=+-|
  Out1 : Outport
  wires:
  Gain/1 -> Sum5/2, Sum7/2, Delay/1
  Delay/1 -> Delay4/1, Sum5/1, Sum7/1
  Delay2/1 -> Sum2/1
  Sum5/1 -> Sum3/2
  Sum6/1 -> Sum4/2
  Sum7/1 -> Sum6/2
  Delay3/1 -> Sum8/1, Sum4/1
  Delay1/1 -> Sum5/3, Delay2/1
  Sum8/1 -> Sum1/1
  In3/1 -> Product1/2, Product/2
  Sum3/1 -> Sum8/2
  Product1/1 -> Sum2/2
  Sum4/1 -> Product/1
  Delay4/1 -> Delay3/1, Sum3/1, Sum6/1
  Sum1/1 -> Product1/1
  Product/1 -> Sum1/2
  i/1 -> Delay1/1, Gain/1
  Sum2/1 -> Out1/1

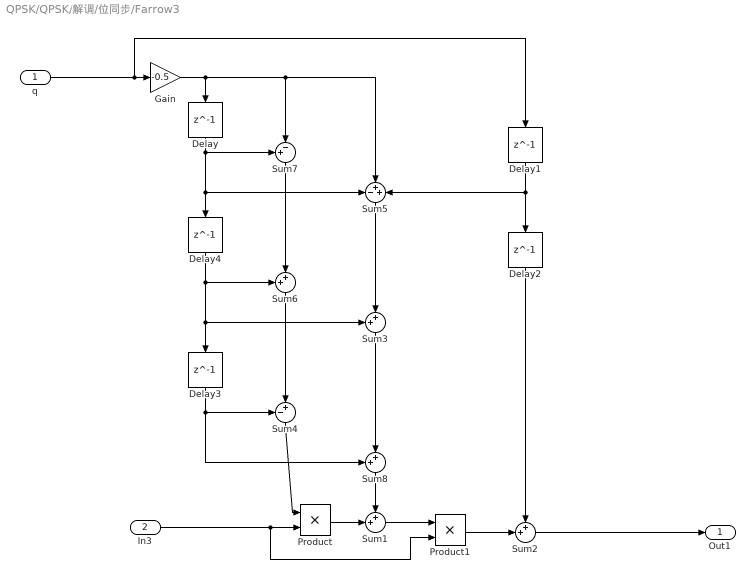
== system QPSK/QPSK/解调/位同步/Farrow3 ==
  q : Inport
  In3 : Inport  Port=2
  Delay{,1..4} (5 alike) : Delay  DelayLength=1  InitialCondition=0
  Gain : Gain  Gain=-0.5  OutDataTypeStr=fixdt(1,32,28)
  Product : Product  OutDataTypeStr=fixdt(1,32,28)
  Product1 : Product  OutDataTypeStr=fixdt(1,32,28)
  Sum{1,3,6,8} (4 alike) : Sum  Inputs=++|
  Sum2 : Sum  Inputs=++|  OutDataTypeStr=fixdt(1,32,28)
  Sum4 : Sum  Inputs=-+|
  Sum5 : Sum  Inputs=-++
  Sum7 : Sum  Inputs=+-|
  Out1 : Outport
  wires:
  Gain/1 -> Sum5/2, Sum7/2, Delay/1
  Delay/1 -> Delay4/1, Sum5/1, Sum7/1
  Delay2/1 -> Sum2/1
  Sum5/1 -> Sum3/2
  Sum6/1 -> Sum4/2
  Sum7/1 -> Sum6/2
  Delay3/1 -> Sum8/1, Sum4/1
  Delay1/1 -> Sum5/3, Delay2/1
  Sum8/1 -> Sum1/1
  In3/1 -> Product1/2, Product/2
  Sum3/1 -> Sum8/2
  Product1/1 -> Sum2/2
  Sum4/1 -> Product/1
  Delay4/1 -> Delay3/1, Sum3/1, Sum6/1
  Sum1/1 -> Product1/1
  Product/1 -> Sum1/2
  q/1 -> Delay1/1, Gain/1
  Sum2/1 -> Out1/1

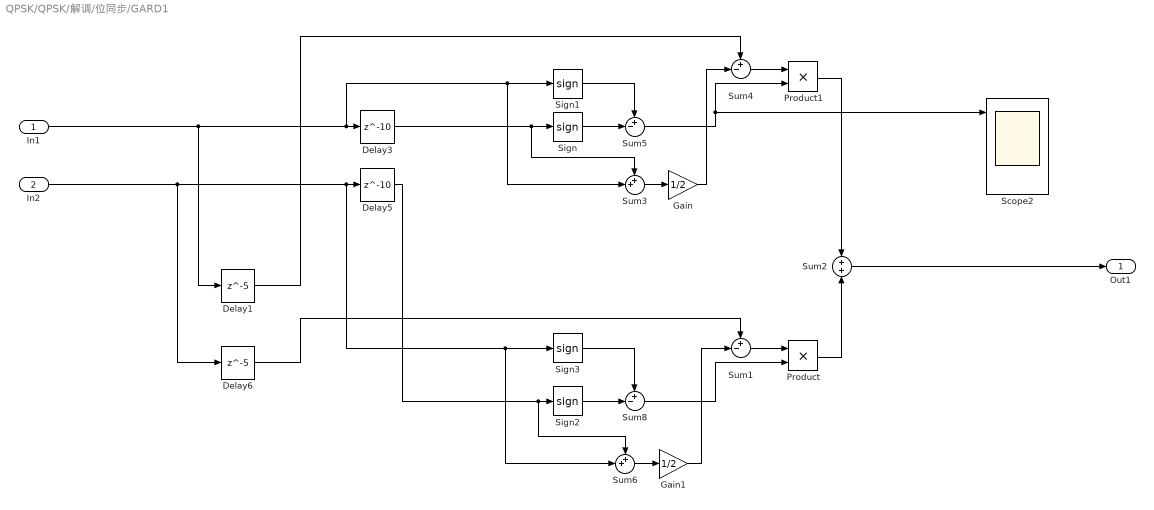
== system QPSK/QPSK/解调/位同步/GARD1 ==
  In1 : Inport
  In2 : Inport  Port=2
  Delay1 : Delay  DelayLength=5  InitialCondition=0
  Delay3 : Delay  DelayLength=10  InitialCondition=0
  Delay5 : Delay  DelayLength=10  InitialCondition=0
  Delay6 : Delay  DelayLength=5  InitialCondition=0
  Gain : Gain  Gain=1/2  OutDataTypeStr=fixdt(1,32,28)
  Gain1 : Gain  Gain=1/2  OutDataTypeStr=fixdt(1,32,28)
  Product : Product  OutDataTypeStr=fixdt(1,32,28)
  Product1 : Product  OutDataTypeStr=fixdt(1,32,28)
  Scope2 : Scope  NumInputPorts=3
  Sign{,1..3} (4 alike) : Signum
  Sum1 : Sum  Inputs=+-|  OutDataTypeStr=fixdt(1,32,28)
  Sum2 : Sum  Inputs=+|+  OutDataTypeStr=fixdt(1,32,28)
  Sum3 : Sum  Inputs=++|
  Sum4 : Sum  Inputs=+-|  OutDataTypeStr=fixdt(1,32,28)
  Sum5 : Sum  Inputs=+-|
  Sum6 : Sum  Inputs=++|
  Sum8 : Sum  Inputs=+-|
  Out1 : Outport
  wires:
  Sum2/1 -> Out1/1
  Sign1/1 -> Sum5/1
  Product1/1 -> Sum2/1
  Delay3/1 -> Sum3/1, Sign/1
  Product/1 -> Sum2/2
  Sign/1 -> Sum5/2
  Sum8/1 -> Product/2
  In1/1 -> Sum3/2, Sign1/1, Delay3/1, Delay1/1
  Sign3/1 -> Sum8/1
  Sum5/1 -> Scope2/1, Product1/2
  Sign2/1 -> Sum8/2
  Sum3/1 -> Gain/1
  Sum4/1 -> Product1/1
  Gain/1 -> Sum4/2
  Delay1/1 -> Sum4/1
  Sum6/1 -> Gain1/1
  Delay5/1 -> Sum6/1, Sign2/1
  In2/1 -> Sum6/2, Sign3/1, Delay5/1, Delay6/1
  Sum1/1 -> Product/1
  Gain1/1 -> Sum1/2
  Delay6/1 -> Sum1/1

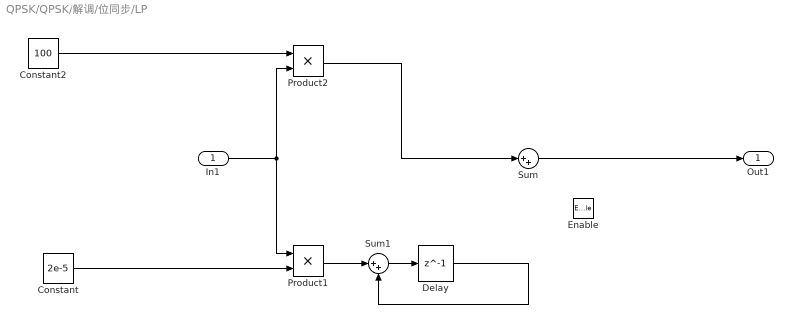
== system QPSK/QPSK/解调/位同步/LP ==
  In1 : Inport
  Enable : EnablePort
  Constant : Constant  Value=2e-5  VectorParams1D=off
  Constant2 : Constant  Value=100  VectorParams1D=off
  Delay : Delay  DelayLength=1  InitialCondition=1
  Product1 : Product  OutDataTypeStr=fixdt(1,64,32)
  Product2 : Product  OutDataTypeStr=fixdt(1,64,32)
  Sum : Sum  Inputs=|++  OutDataTypeStr=fixdt(1,64,32)
  Sum1 : Sum  Inputs=|++  OutDataTypeStr=fixdt(1,64,32)
  Out1 : Outport
  wires:
  In1/1 -> Product1/1, Product2/2
  Product2/1 -> Sum/1
  Product1/1 -> Sum1/1
  Sum1/1 -> Delay/1
  Delay/1 -> Sum1/2
  Constant2/1 -> Product2/1
  Constant/1 -> Product1/2
  Sum/1 -> Out1/1

== system QPSK/QPSK/解调/位同步/Subsystem ==
  In1 : Inport
  In2 : Inport  Port=2
  Enable : EnablePort
  Out1 : Outport
  Out2 : Outport  Port=2
  wires:
  In1/1 -> Out1/1
  In2/1 -> Out2/1

== system QPSK/QPSK/解调/位同步/Subsystem1 ==
  In1 : Inport
  Enable : EnablePort
  Out1 : Outport
  wires:
  In1/1 -> Out1/1

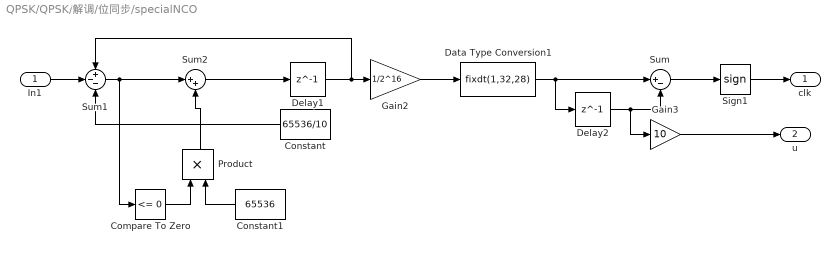
== system QPSK/QPSK/解调/位同步/specialNCO ==
  In1 : Inport
  Compare To Zero : simulink/Logic and Bit Operations/Compare To Zero  relop=<=  OutDataTypeStr=boolean
  Constant : Constant  Value=65536/10
  Constant1 : Constant  Value=65536
  Data Type Conversion1 : DataTypeConversion  OutDataTypeStr=fixdt(1,32,28)
  Delay1 : Delay  DelayLength=1  InitialCondition=0
  Delay2 : Delay  DelayLength=1  InitialCondition=0
  Gain2 : Gain  Gain=1/2^16
  Gain3 : Gain  Gain=10
  Product : Product
  Sign1 : Signum
  Sum : Sum  Inputs=|+-
  Sum1 : Sum  Inputs=+--  OutMin=[0]  OutDataTypeStr=fixdt(1,64,32)
  Sum2 : Sum  Inputs=|++  OutDataTypeStr=fixdt(1,64,32)
  clk : Outport
  u : Outport  Port=2
  wires:
  Delay1/1 -> Sum1/1, Gain2/1
  Sum/1 -> Sign1/1
  Sign1/1 -> clk/1
  Gain2/1 -> Data Type Conversion1/1
  Gain3/1 -> u/1
  In1/1 -> Sum1/2
  Constant/1 -> Sum1/3
  Delay2/1 -> Gain3/1, Sum/2
  Data Type Conversion1/1 -> Sum/1, Delay2/1
  Sum1/1 -> Sum2/1, Compare To Zero/1
  Sum2/1 -> Delay1/1
  Constant1/1 -> Product/2
  Compare To Zero/1 -> Product/1
  Product/1 -> Sum2/2

== system QPSK/QPSK/解调/载波同步/LP ==
  In1 : Inport
  Constant : Constant  Value=2e-2  VectorParams1D=off
  Constant2 : Constant  Value=10  VectorParams1D=off
  Delay : Delay  DelayLength=1  InitialCondition=0.1
  Product1 : Product  OutDataTypeStr=fixdt(1,32,15)
  Product2 : Product  OutDataTypeStr=fixdt(1,32,15)
  Sum : Sum  Inputs=|++  OutDataTypeStr=fixdt(1,32,15)
  Sum1 : Sum  Inputs=|++  OutDataTypeStr=fixdt(1,32,15)
  Out1 : Outport
  wires:
  In1/1 -> Product1/1, Product2/2
  Product2/1 -> Sum/1
  Product1/1 -> Sum1/1
  Sum1/1 -> Delay/1
  Delay/1 -> Sum/2, Sum1/2
  Constant2/1 -> Product2/1
  Constant/1 -> Product1/2
  Sum/1 -> Out1/1
